simulink model "ASK"  (R2013a)
settings: Solver=ode45  StartTime=0.0  StopTime=100  RelTol=1e-3
libraries: commchan3 x1, commrandsrc2 x1, commsink2 x1
settings Model: Creator=Fred  LastModifiedBy=Fred

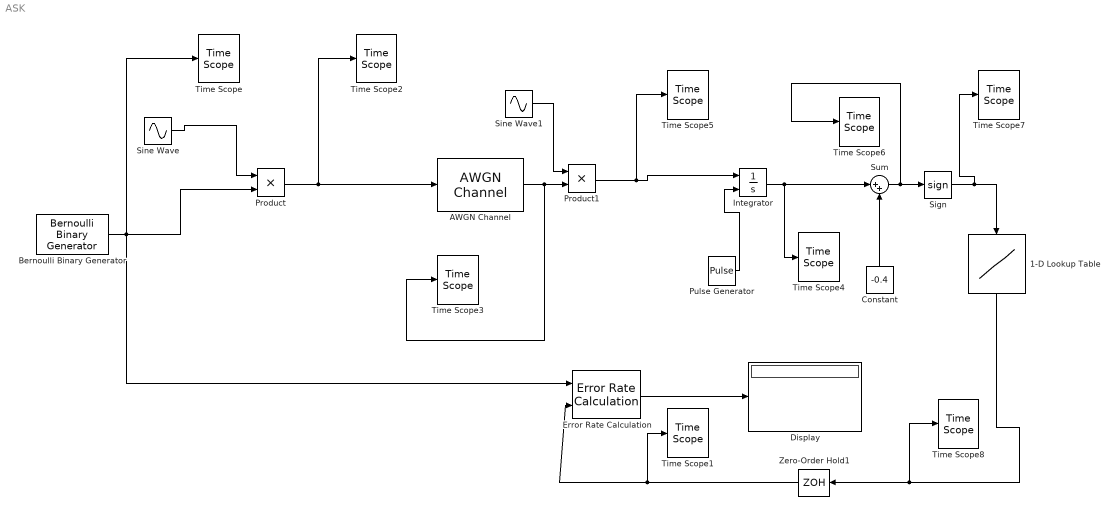
== system ASK ==
  1-D Lookup Table : Lookup_n-D  NumberOfTableDimensions=1  BreakpointsForDimension1=[-1:1]  Table=[0,0,1]  RndMeth=Simplest  InputSameDT=on
  AWGN Channel : commchan3/AWGN Channel  InputProcessing=Inherited (this choice will be removed - see release notes)  seed=67  noiseMode=Variance from mask  EbNodB=10  EsNodB=10  SNRdB=10  bitsPerSym=1  Ps=1  Tsym=1  variance=1
  Bernoulli Binary Generator : commrandsrc2/Bernoulli Binary Generator  P=0.5  seed=61  Ts=1  frameBased=off  sampPerFrame=1  orient=off  outDataType=double
  Constant : Constant  Value=-0.4
  Display : Display
      settings: Decimation=9
  Error Rate Calculation : commsink2/Error Rate Calculation  N=1  st_delay=0  cp_mode=Entire frame  subframe=[]  PMode=Port  WsName=ErrorVec  RsMode2=off  stop=off  numErr=100  maxBits=1e6
  Integrator : Integrator  ExternalReset=rising
  Product : Product
  Product1 : Product  OutDataTypeStr=double
  Pulse Generator : DiscretePulseGenerator  PulseType=Time based  Period=1  PulseWidth=50  PhaseDelay=1.01
  Sign : Signum
  Sine Wave : Sin  Frequency=10*pi  SampleTime=0.01
  Sine Wave1 : Sin  Frequency=10*pi  SampleTime=0.01
  Sum : Sum  Inputs=|++
  Time Scope{,1..8} (9 alike) : TimeScope  DefaultConfigurationName=spbscopes.TimeScopeBlockCfg
      settings: CopyFcn=scopeextensions.ScopeBlock.callback(gcbh, 'onBlockCopy', gcbh);  DeleteFcn=scopeextensions.ScopeBlock.callback(gcbh, 'onBlockDelete');  PreSaveFcn=scopeextensions.ScopeBlock.callback(gcbh, 'onModelSave');  NameChangeFcn=scopeextensions.ScopeBlock.callback(gcbh, 'onBlockRename');  CloseFcn=scopeextensions.ScopeBlock.callback(gcbh, 'onBlockClose');  PreDeleteFcn=scopeextensions.ScopeBlock.callback(gcbh, 'onBlockPreDelete');
  Zero-Order Hold1 : ZeroOrderHold
  wires:
  Constant/1 -> Sum/2
  AWGN Channel/1 -> Time Scope3/1, Product1/2
  Sine Wave1/1 -> Product1/1
  Product/1 -> Time Scope2/1, AWGN Channel/1
  Product1/1 -> Time Scope5/1, Integrator/1
  Sign/1 -> Time Scope7/1, 1-D Lookup Table/1
  Error Rate Calculation/1 -> Display/1
  1-D Lookup Table/1 -> Time Scope8/1, Zero-Order Hold1/1
  Bernoulli Binary Generator/1 -> Error Rate Calculation/1, Time Scope/1, Product/2
  Pulse Generator/1 -> Integrator/2
  Sine Wave/1 -> Product/1
  Zero-Order Hold1/1 -> Time Scope1/1, Error Rate Calculation/2
  Integrator/1 -> Time Scope4/1, Sum/1
  Sum/1 -> Time Scope6/1, Sign/1
